simulink model "InnerOuter_Sim"  (Simulink 6.6)
settings: Solver=ode4  StartTime=0.0  StopTime=125  FixedStep=SampleT  RelTol=1e-3
InitFcn:
  | clc
  | innerOuterInit
undefined symbols (not defined in the file): A1, Apolar, apSampleTime, bankCommandLimit, baseHeight, baseTemp, CD0, chord, CL0, CLa, CLa_dot, Clb, ClDa, CLDe, CLDf, ClDr, clock, Clp, CLq, Clr, Cm0, Cma, CmDe, CmDf, Cmq, Cnb, CnDa, CnDr, Cnp, Cnr, compensatorOn, CYb, CYDr, da_failamp, da_failbias, da_failper, daL_fail, daLimit, daR_fail, deg, deLimit, derivativesConstant, dr_fail, dr_failamp, dr_failbias, dr_failper, drLimit, dtLimit, Earth, elarm, Euler_0, F, gaind, getWP, ISA_g, Ixx, Iyy, Izz, L1OF, L2_base ... (+28)
libraries: simulink x102, SLUGS_Library x23, aerolibconvert2 x15, dsPICdrivers x8, aerolibactuator x5, aerolibtransform2 x2, aerolibwind2 x2, dspmtrx3 x2, aerolibatmos2 x1, aerolibutil x1
(part 2 of 4)

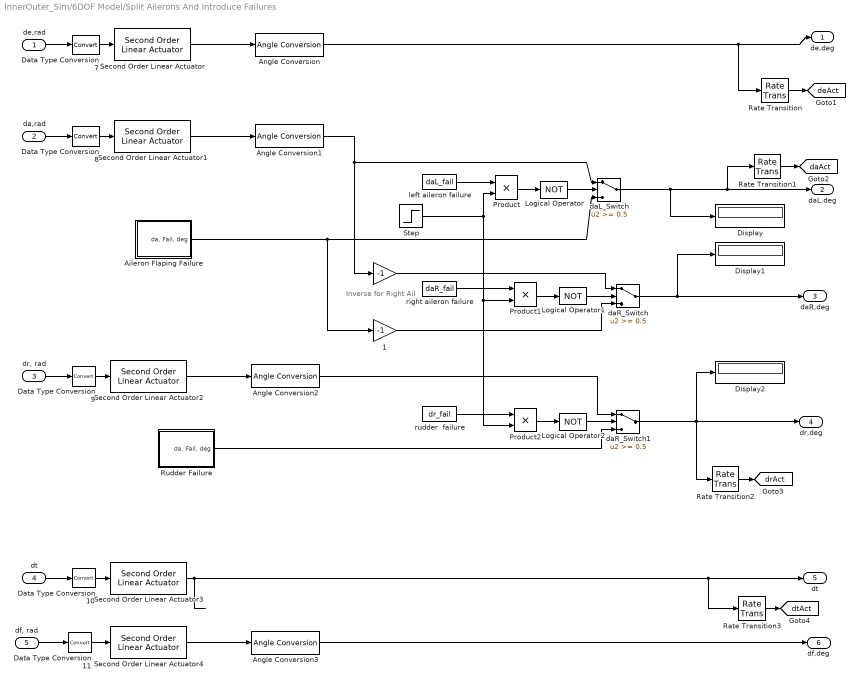
== system InnerOuter_Sim/6DOF Model/Split Ailerons And Introduce Failures ==
  note: Inverse
      | for Right
      | Ail
  de,rad : Inport
  da,rad : Inport  Port=2
  "dr, rad" : Inport  Port=3
  dt : Inport  Port=4
  "df, rad" : Inport  Port=5
  " " : Gain  Gain=-1  SaturateOnIntegerOverflow=on
  " 1" : Gain  Gain=-1  SaturateOnIntegerOverflow=on
  Aileron Flaping Failure : Subsystem
  Angle Conversion{,1..3} (4 alike) : aerolibconvert2/Angle Conversion  SystemSampleTime=-1  IU=rad  OU=deg
  Data Type Conversion{7..11} (5 alike) : DataTypeConversion  OutDataTypeMode=double
  Display : Display
  Display1 : Display
  Display2 : Display
  Logical Operator : Logic  Operator=NOT  AllPortsSameDT=off  OutDataTypeMode=Boolean
  Logical Operator1 : Logic  Operator=NOT  AllPortsSameDT=off  OutDataTypeMode=Boolean
  Logical Operator2 : Logic  Operator=NOT  AllPortsSameDT=off  OutDataTypeMode=Boolean
  Product : Product  RndMeth=Zero
  Product1 : Product  RndMeth=Zero
  Product2 : Product  RndMeth=Zero
  Rate Transition{,1..3} (4 alike) : RateTransition  OutPortSampleTime=apSampleTime
  Rudder Failure : Subsystem
  Second Order Linear Actuator{,1..3} (4 alike) : aerolibactuator/Second Order Linear Actuator  SystemSampleTime=-1  wn_fin=15  z_fin=0.8  fin_act_0=0
  Second Order Linear Actuator4 : aerolibactuator/Second Order Linear Actuator  SystemSampleTime=-1  wn_fin=150  z_fin=0.7  fin_act_0=0
  Step : Step  Time=tfailure
  daL_Switch : Switch  Threshold=0.5
  daR_Switch : Switch  Threshold=0.5
  daR_Switch1 : Switch  Threshold=0.5
  left aileron failure : Constant  Value=daL_fail
  right aileron failure : Constant  Value=daR_fail
  rudder  failure : Constant  Value=dr_fail
  de,deg : Outport
  daL,deg : Outport  Port=2
  daR,deg : Outport  Port=3
  dr,deg : Outport  Port=4
  "dt " : Outport  Port=5
  df,deg : Outport  Port=6
  tag scope: daAct=global, deAct=global, drAct=global, dtAct=global
  wires:
  de,rad/1 -> Data Type Conversion7/1
  da,rad/1 -> Data Type Conversion8/1
  "dr, rad"/1 -> Data Type Conversion9/1
  dt/1 -> Data Type Conversion10/1
  "df, rad"/1 -> Data Type Conversion11/1
  Second Order Linear Actuator/1 -> Angle Conversion/1
  Second Order Linear Actuator1/1 -> Angle Conversion1/1
  Second Order Linear Actuator2/1 -> Angle Conversion2/1
  Second Order Linear Actuator3/1 -> "dt "/1, Rate Transition3/1
  Second Order Linear Actuator4/1 -> Angle Conversion3/1
  Rate Transition1/1 -> [daAct]
  Rate Transition2/1 -> [drAct]
  Rate Transition3/1 -> [dtAct]
  Data Type Conversion7/1 -> Second Order Linear Actuator/1
  Data Type Conversion8/1 -> Second Order Linear Actuator1/1
  Data Type Conversion9/1 -> Second Order Linear Actuator2/1
  Data Type Conversion10/1 -> Second Order Linear Actuator3/1
  Data Type Conversion11/1 -> Second Order Linear Actuator4/1
  Angle Conversion/1 -> de,deg/1, Rate Transition/1
  Angle Conversion1/1 -> daL_Switch/1, " "/1
  Angle Conversion2/1 -> daR_Switch1/1
  Angle Conversion3/1 -> df,deg/1
  left aileron failure/1 -> Product/1
  Aileron Flaping Failure/1("da, Fail, deg") -> daL_Switch/3, " 1"/1
  Product/1 -> Logical Operator/1
  Logical Operator/1 -> daL_Switch/2
  Step/1 -> Product/2, Product1/2, Product2/2
  daL_Switch/1 -> Display/1, daL,deg/1, Rate Transition1/1
  right aileron failure/1 -> Product1/1
  Product1/1 -> Logical Operator1/1
  Logical Operator1/1 -> daR_Switch/2
  " "/1 -> daR_Switch/1
  " 1"/1 -> daR_Switch/3
  daR_Switch/1 -> daR,deg/1, Display1/1
  rudder  failure/1 -> Product2/1
  Product2/1 -> Logical Operator2/1
  Logical Operator2/1 -> daR_Switch1/2
  daR_Switch1/1 -> dr,deg/1, Display2/1, Rate Transition2/1
  Rate Transition/1 -> [deAct]
  Rudder Failure/1("da, Fail, deg") -> daR_Switch1/3

== system InnerOuter_Sim/6DOF Model/Subsystem ==
  Signal In : Inport  Orientation=down
  Noise On : Inport  Port=2
  Add : Sum  OutScaling=2^-10
  Random Number : RandomNumber  Variance=nv  Seed=ns  SampleTime=st
  Signal1 : InportShadow  Port=1  LatchByCopyingInsideSignal=off
  Switch : Switch  Threshold=0.3
  Signal Out : Outport
  wires:
  Random Number/1 -> Add/2
  Add/1 -> Switch/1
  Signal In/1 -> Add/1
  Noise On/1 -> Switch/2
  Switch/1 -> Signal Out/1
  Signal1/1 -> Switch/3

== system InnerOuter_Sim/6DOF Model/Subsystem1 ==
  Signal In : Inport  Orientation=down
  Noise On : Inport  Port=2
  Add : Sum  OutScaling=2^-10
  Random Number : RandomNumber  Variance=nv  Seed=ns  SampleTime=st
  Signal1 : InportShadow  Port=1  LatchByCopyingInsideSignal=off
  Switch : Switch  Threshold=0.3
  Signal Out : Outport
  wires:
  Signal1/1 -> Switch/3
  Switch/1 -> Signal Out/1
  Noise On/1 -> Switch/2
  Signal In/1 -> Add/1
  Add/1 -> Switch/1
  Random Number/1 -> Add/2

== system InnerOuter_Sim/6DOF Model/Subsystem2 ==
  Signal In : Inport  Orientation=down
  Noise On : Inport  Port=2
  Add : Sum  OutScaling=2^-10
  Random Number : RandomNumber  Variance=nv  Seed=ns  SampleTime=st
  Signal1 : InportShadow  Port=1  LatchByCopyingInsideSignal=off
  Switch : Switch  Threshold=0.3
  Signal Out : Outport
  wires:
  Random Number/1 -> Add/2
  Add/1 -> Switch/1
  Signal In/1 -> Add/1
  Noise On/1 -> Switch/2
  Switch/1 -> Signal Out/1
  Signal1/1 -> Switch/3

== system InnerOuter_Sim/6DOF Model/Subsystem3 ==
  Signal In : Inport  Orientation=down
  Noise On : Inport  Port=2
  Add : Sum  OutScaling=2^-10
  Random Number : RandomNumber  Variance=nv  Seed=ns  SampleTime=st
  Signal1 : InportShadow  Port=1  LatchByCopyingInsideSignal=off
  Switch : Switch  Threshold=0.3
  Signal Out : Outport
  wires:
  Signal1/1 -> Switch/3
  Switch/1 -> Signal Out/1
  Noise On/1 -> Switch/2
  Signal In/1 -> Add/1
  Add/1 -> Switch/1
  Random Number/1 -> Add/2

== system InnerOuter_Sim/6DOF Model/Subsystem4 ==
  Signal In : Inport  Orientation=down
  Noise On : Inport  Port=2
  Add : Sum  OutScaling=2^-10
  Random Number : RandomNumber  Variance=nv  Seed=ns  SampleTime=st
  Signal1 : InportShadow  Port=1  LatchByCopyingInsideSignal=off
  Switch : Switch  Threshold=0.3
  Signal Out : Outport
  wires:
  Signal1/1 -> Switch/3
  Switch/1 -> Signal Out/1
  Noise On/1 -> Switch/2
  Signal In/1 -> Add/1
  Add/1 -> Switch/1
  Random Number/1 -> Add/2

== system InnerOuter_Sim/6DOF Model/Subsystem5 ==
  Signal In : Inport  Orientation=down
  Noise On : Inport  Port=2
  Add : Sum  OutScaling=2^-10
  Random Number : RandomNumber  Variance=nv  Seed=ns  SampleTime=st
  Signal1 : InportShadow  Port=1  LatchByCopyingInsideSignal=off
  Switch : Switch  Threshold=0.3
  Signal Out : Outport
  wires:
  Random Number/1 -> Add/2
  Add/1 -> Switch/1
  Signal In/1 -> Add/1
  Noise On/1 -> Switch/2
  Switch/1 -> Signal Out/1
  Signal1/1 -> Switch/3

== system InnerOuter_Sim/6DOF Model/Subsystem6 ==
  Signal In : Inport  Orientation=down
  Noise On : Inport  Port=2
  Add : Sum  OutScaling=2^-10
  Random Number : RandomNumber  Variance=nv  Seed=ns  SampleTime=st
  Signal1 : InportShadow  Port=1  LatchByCopyingInsideSignal=off
  Switch : Switch  Threshold=0.3
  Signal Out : Outport
  wires:
  Signal1/1 -> Switch/3
  Switch/1 -> Signal Out/1
  Noise On/1 -> Switch/2
  Signal In/1 -> Add/1
  Add/1 -> Switch/1
  Random Number/1 -> Add/2

== system InnerOuter_Sim/BaroTest/Compute Barometric Height ==
  Base Height (m) : Inport
  Base Pressure (Pa) : Inport  Port=2
  Baro (Pa) : Inport  Port=3
  Constant2 : Constant  Value=baseTemp/(-LapseRate)  OutDataTypeMode=single
  Constant3 : Constant  Value=9.350253e-2  OutDataTypeMode=single
  Constant4 : Constant  Value=-1.888933e-1  OutDataTypeMode=single
  Constant5 : Constant  Value=2.180313e-5  OutDataTypeMode=single
  Divide : Product  Inputs=*/  OutDataTypeMode=single  OutScaling=2^-10
  Divide{1..4} (4 alike) : Product  OutDataTypeMode=single  OutScaling=2^-10
  Length Conversion : aerolibconvert2/Length Conversion  SystemSampleTime=-1  IU=ft  OU=m
  Sum1 : Sum  Inputs=|++  OutDataTypeMode=single
  Sum2 : Sum  Inputs=|+-  OutDataTypeMode=single
  Sum3 : Sum  Inputs=3  OutDataTypeMode=single
  "Altitude, m" : Outport
  wires:
  Length Conversion/1 -> Sum1/1
  Sum2/1 -> Divide/1
  Sum1/1 -> "Altitude, m"/1
  Divide3/1 -> Length Conversion/1
  Constant2/1 -> Divide3/2
  Sum3/1 -> Divide3/1
  Constant5/1 -> Sum3/3
  Divide2/1 -> Sum3/2
  Divide1/1 -> Sum3/1
  Constant4/1 -> Divide2/2
  Constant3/1 -> Divide1/2
  Divide4/1 -> Divide1/1  "x^2"
  Divide/1 -> Divide2/1, Divide4/1, Divide4/2  "x"
  Base Pressure (Pa)/1 -> Divide/2, Sum2/2
  Base Height (m)/1 -> Sum1/2
  Baro (Pa)/1 -> Sum2/1

== system InnerOuter_Sim/BaroTest/Initial Baro Bias ==
  Baro (Pa) : Inport
  Enable : EnablePort
  Data Type Conversion : DataTypeConversion  OutDataTypeMode=double
  Data Type Conversion1 : DataTypeConversion  OutDataTypeMode=single
  Low Pass8 : Subsystem  mask(DiscretizedZeroPole){Zeros=[], Poles=[-3], Gain=3, AbsTol=auto, SampleTime=.01, method=tustin, Wc=1}
      mask prompts: Zeros "Zeros (enter in s-main:)"; Poles "Poles (enter in s-domain:)"; Gain "Gain (enter in s-domain:)"; AbsTol "Absolute tolerance:"; SampleTime "Sample time:"; Wc "Critical Frequency (Hz):"
      mask help: Continuous mask uses c2d to transform parameters onto the Discrete Zero-Pole block inside.
      mask init:
      | st=SampleTime;
      | if length(st)>1
      |     st=SampleTime(1);
      | end
      | if(st>0)
      |     [zerosd,polesd,gaind] = sldiscutil('disczpk', {st,method,Wc,Zeros,Poles,Gain});
      | end	
      | s = get_param(gcb,'maskvalues');
      | zeross = s{1};
      | poless = s{2};
      | gainss = s{3};
      | %zerosc = eval(zeross);
      | %polesc = eval(poless);
      | %gainsc = eval(gainss);
      | sldiscutil('initzpkmask', st);
      | if(st==0)
      | set_param([gcb '/Zero Pole'], 'AbsoluteTolerance', AbsTol);
      | end
      mask StyleString: edit,edit,edit,edit,edit,popup(zoh|foh|tustin|prewarp|matched),edit
      mask CallbackString: |||||hidecrit|
      mask Display:
      | droots(zeross,poless,gainss)
      | text( 0.5, 1.0, method, 'verticalAlignment','top')
  Mux : Mux  Inputs=2
  Scope : Scope
      settings: SaveName=ScopeData8
  "[80k - 120k]" : Saturate  UpperLimit=120000  LowerLimit=80000
  Baro (Gnd) : Outport
  wires:
  Baro (Pa)/1 -> Data Type Conversion/1
  Low Pass8/1(Out1) -> Data Type Conversion1/1
  Data Type Conversion/1 -> Low Pass8/1(In1)
  Data Type Conversion1/1 -> Mux/2, "[80k - 120k]"/1
  Mux/1 -> Scope/1
  "[80k - 120k]"/1 -> Baro (Gnd)/1, Mux/1

== system InnerOuter_Sim/BaroTest/Zero Out Height ==
  Base Height : Inport
  Computed Height : Inport  Port=2
  Enable : EnablePort
  Integer Delay : simulink/Discrete/Integer Delay  vinit=0  samptime=.01  NumDelays=1
  Sum : Sum  Inputs=|+-  OutDataTypeMode=single
  Height Offset : Outport
  wires:
  Computed Height/1 -> Integer Delay/1
  Sum/1 -> Height Offset/1
  Integer Delay/1 -> Sum/2
  Base Height/1 -> Sum/1

== system InnerOuter_Sim/Compute psi_dot_m/Subsystem5 ==
  u : Inport
  C Function Call1 : dsPICdrivers/OTHERS/C Function Call  Tag=dsPIC_dsPIC_CFunctionCall  fctName='myCos'  INPUT_SIZE=1  INPUT1=real32  INPUT2=--  INPUT3=--  OUTPUT_SIZE=1  OUTPUT1=real32  SampleTime=-1  InputType=[ 7 ]  OutputType=[ 7 ]  FctDeclaration=extern real32_T myCos(real32_T u1);  FctCall=%y1 = myCos(%u1);  OrderingInOutPopup=None
  Environment Controller1 : simulink/Signal Routing/Environment Controller  SystemSampleTime=-1
  Trigonometric Function : Trigonometry  Operator=cos
  cos(u) : Outport
  wires:
  u/1 -> C Function Call1/1, Trigonometric Function/1
  Environment Controller1/1 -> cos(u)/1
  C Function Call1/1 -> Environment Controller1/2
  Trigonometric Function/1 -> Environment Controller1/1

== system InnerOuter_Sim/L1 Output Feedback Controller With  Projection Operator/Control  Law ==
  a : Inport
  u : Inport  Port=2
  Compute Coef : Subsystem
  Detect Change : Subsystem
  Divide : Product  OutScaling=2^-10  SampleTime=apSampleTime
  Divide1 : Product  OutScaling=2^-10  SampleTime=apSampleTime
  IC : InitialCondition
  Integer Delay : simulink/Discrete/Integer Delay  vinit=0.0  samptime=apSampleTime  NumDelays=1
  Integer Delay1 : simulink/Discrete/Integer Delay  Orientation=left  vinit=0.0  samptime=apSampleTime  NumDelays=1
  Subtract : Sum  OutScaling=2^-10  SampleTime=apSampleTime
  y : Outport
  wires:
  Integer Delay1/1 -> Divide1/2
  u/1 -> Integer Delay/1
  IC/1 -> Compute Coef/Enable
  Subtract/1 -> Integer Delay1/1, y/1
  Divide1/1 -> Subtract/2
  Divide/1 -> Subtract/1
  Integer Delay/1 -> Divide/2
  Detect Change/1(change?) -> IC/1
  Compute Coef/2(c) -> Divide1/1
  Compute Coef/1(b) -> Divide/1
  a/1 -> Detect Change/1(Data), Compute Coef/1(a)

== system InnerOuter_Sim/L1 Output Feedback Controller With  Projection Operator/Projection Operator ==
  Theta Max : Inport
  Eps 0 : Inport  Port=2
  Theta : Inport  Port=3
  y : Inport  Port=4
  Compare To Zero : simulink/Logic and Bit Operations/Compare To Zero  SystemSampleTime=-1  relop=>=  LogicOutDataTypeMode=boolean  ZeroCross=off
  Compare To Zero1 : simulink/Logic and Bit Operations/Compare To Zero  SystemSampleTime=-1  relop=>  LogicOutDataTypeMode=boolean  ZeroCross=off
  Data Type Conversion1 : DataTypeConversion  OutDataType=fixdt(1, 16)
  Divide2 : Product  OutDataTypeMode=single  OutScaling=2^-10
  Enabled Subsystem : Subsystem  TreatAsAtomicUnit=on
  Enabled Subsystem1 : Subsystem  TreatAsAtomicUnit=on
  Enabled Subsystem2 : Subsystem  TreatAsAtomicUnit=on
  F(theta) : Subsystem
  Logical Operator : Logic  Operator=NOT  AllPortsSameDT=off  OutDataTypeMode=Specify via dialog
  Logical Operator2 : Logic  Orientation=down  AllPortsSameDT=off  OutDataTypeMode=Specify via dialog
  Merge : Merge  InitialOutput=0
  Scope1 : Scope  NumInputPorts=4
      settings: YMin=-0.6~-0.5~-100~-10  YMax=0~5~10~10  SaveName=ScopeData4
  Scope2 : Scope  NumInputPorts=2
      settings: TimeRange=400  YMin=-0.06~-0.06  YMax=0.06~0.06  SaveName=ScopeData15
  "y " : InportShadow  Port=4  LatchByCopyingInsideSignal=off
  "y    " : InportShadow  Port=4  LatchByCopyingInsideSignal=off
  "Proj(the, y)" : Outport
  wires:
  Enabled Subsystem1/1(Out1) -> Merge/2
  "y    "/1 -> Enabled Subsystem1/1(y), Enabled Subsystem2/1(y), Scope1/2
  Logical Operator/1 -> Enabled Subsystem/Enable, Scope2/2
  Logical Operator2/1 -> Logical Operator/1, Enabled Subsystem1/Enable, Enabled Subsystem2/Enable, Scope2/1
  Compare To Zero1/1 -> Logical Operator2/1
  F(theta)/2(dif_f_theta) -> Divide2/1, Enabled Subsystem1/3(grad), Enabled Subsystem2/3(grad), Scope1/4
  Compare To Zero/1 -> Logical Operator2/2
  Enabled Subsystem/1(Out1) -> Data Type Conversion1/1
  "y "/1 -> Enabled Subsystem/1(In1)
  Merge/1 -> "Proj(the, y)"/1
  Divide2/1 -> Compare To Zero1/1
  y/1 -> Divide2/2
  F(theta)/1(f_theta) -> Compare To Zero/1, Enabled Subsystem1/2(f_the), Enabled Subsystem2/2(f_the), Scope1/3
  Theta/1 -> F(theta)/3(Theta)
  Eps 0/1 -> F(theta)/2(Eps 0)
  Theta Max/1 -> F(theta)/1(Theta Max)
  Data Type Conversion1/1 -> Merge/1
  Enabled Subsystem2/1(Out1) -> Scope1/1

== system InnerOuter_Sim/L1 Output Feedback Controller With  Projection Operator/State Predictor ==
  a : Inport
  u : Inport  Port=2
  Compute Coef : Subsystem
  Detect Change : Subsystem
  Divide : Product  OutScaling=2^-10  SampleTime=apSampleTime
  Divide1 : Product  OutScaling=2^-10  SampleTime=apSampleTime
  IC : InitialCondition
  Integer Delay : simulink/Discrete/Integer Delay  vinit=0.0  samptime=apSampleTime  NumDelays=1
  Integer Delay1 : simulink/Discrete/Integer Delay  Orientation=left  vinit=0.0  samptime=apSampleTime  NumDelays=1
  Subtract : Sum  OutScaling=2^-10  SampleTime=apSampleTime
  y : Outport
  wires:
  a/1 -> Compute Coef/1(a), Detect Change/1(Data)
  Compute Coef/1(b) -> Divide/1
  Compute Coef/2(c) -> Divide1/1
  Detect Change/1(change?) -> IC/1
  Integer Delay/1 -> Divide/2
  Divide/1 -> Subtract/1
  Divide1/1 -> Subtract/2
  Subtract/1 -> y/1, Integer Delay1/1
  IC/1 -> Compute Coef/Enable
  u/1 -> Integer Delay/1
  Integer Delay1/1 -> Divide1/2

== system InnerOuter_Sim/L1 Output Feedback Controller With  Projection Operator/Trapezoidal Integrator ==
  x : Inport
  Reset : Inport  Port=2
  Constant : Constant  Value=1/3  OutDataTypeMode=single
  Constant1 : Constant  Value=4/3  OutDataTypeMode=single
  Constant2 : Constant  Value=T/2  OutDataTypeMode=single
  Constant3 : Constant  Value=1/3  OutDataTypeMode=single
  Constant5 : Constant  Orientation=left  Value=0  OutDataTypeMode=single
  Integer Delay : simulink/Discrete/Integer Delay  vinit=0.0  samptime=T  NumDelays=1
  Integer Delay1 : simulink/Discrete/Integer Delay  vinit=0.0  samptime=T  NumDelays=2
  Integer Delay2 : simulink/Discrete/Integer Delay  Orientation=left  vinit=0.0  samptime=T  NumDelays=1
  Product{,1..3} (4 alike) : Product  OutDataTypeMode=single  RndMeth=Zero
  Protect NaNs : Subsystem
  Protect NaNs1 : Subsystem
  Subtract : Sum  Inputs=3  OutDataTypeMode=single  OutScaling=2^-10
  Subtract1 : Sum  Inputs=2  OutDataTypeMode=single  OutScaling=2^-10
  Switch1 : Switch  Criteria=u2 > Threshold  Threshold=0.3  SampleTime=.01
  "[min max]" : Saturate  UpperLimit=upperLimit  LowerLimit=lowerLimit  SampleTime=T
  Int(x) : Outport
  wires:
  Protect NaNs1/1(Out1) -> Integer Delay2/1, Int(x)/1
  Protect NaNs/1(Out1) -> Integer Delay1/1, Integer Delay/1, Product/1
  Subtract1/1 -> "[min max]"/1
  Product3/1 -> Subtract1/2
  "[min max]"/1 -> Switch1/3
  Switch1/1 -> Protect NaNs1/1(In1)
  Reset/1 -> Switch1/2
  Constant5/1 -> Switch1/1
  Integer Delay2/1 -> Subtract1/1
  Subtract/1 -> Product3/2
  Constant2/1 -> Product3/1
  Product2/1 -> Subtract/3
  Product1/1 -> Subtract/2
  Product/1 -> Subtract/1
  x/1 -> Protect NaNs/1(In1)
  Constant3/1 -> Product2/2
  Integer Delay1/1 -> Product2/1
  Integer Delay/1 -> Product1/1
  Constant1/1 -> Product1/2
  Constant/1 -> Product/2

== system InnerOuter_Sim/Lateral Channel/0.5 sec  tau ==
  In1 : Inport
  Constant : Constant  Value=T
  Constant1 : Constant  Value=f
  Embedded MATLAB Function : Stateflow chart
  Out1 : Outport
  wires:
  In1/1 -> Embedded MATLAB Function/1(u)
  Embedded MATLAB Function/1(y) -> Out1/1
  Constant1/1 -> Embedded MATLAB Function/3(f)
  Constant/1 -> Embedded MATLAB Function/2(T)

== system InnerOuter_Sim/Lateral Channel/Bank to Psi Dot ==
  phi_c : Inport
  U_m : Inport  Port=2
  Constant1 : Constant  Value=9.80665  OutDataTypeMode=single
  Divide : Product  Inputs=/*  OutDataTypeMode=single  OutScaling=2^-10  SampleTime=apSampleTime
  Divide1 : Product  OutDataTypeMode=single  OutScaling=2^-10  SampleTime=apSampleTime
  Subsystem8 : SLUGS_Library/Subsystem8  SystemSampleTime=-1
  negprotect : Stateflow chart
  psi_dot_c : Outport
  wires:
  negprotect/1(zpVal) -> Divide/1
  Divide/1 -> Divide1/2
  phi_c/1 -> Subsystem8/1
  Subsystem8/1 -> Divide1/1
  Divide1/1 -> psi_dot_c/1
  Constant1/1 -> Divide/2
  U_m/1 -> negprotect/1(val)

== system InnerOuter_Sim/Lateral Channel/Sideslip Compensation ==
  phi_m : Inport
  r_m : Inport  Port=2
  U_m : Inport  Port=3
  Enable : EnablePort  StatesWhenEnabling=reset
  Bank to Psi Dot : Subsystem  AncestorBlock=SLUGS_Library/Navigation/Bank to Psi Dot
  Constant : Constant  Value=0.3  OutDataTypeMode=single
  Low Pass : Subsystem
      mask Display:
      | droots([],'-a','a')
      | port_label('input',1,'a')
      | port_label('input',2,'u')
      | port_label('output',1,'y')
  Subtract : Sum  Inputs=+-  OutScaling=2^-10
  psi_dot to Bank : Subsystem  AncestorBlock=SLUGS_Library/Navigation/psi_dot to Bank
  bankComp : Outport  OutputWhenDisabled=reset  InitialOutput=0
  wires:
  phi_m/1 -> Bank to Psi Dot/1(phi_c)
  r_m/1 -> Subtract/2
  U_m/1 -> Bank to Psi Dot/2(U_m), psi_dot to Bank/2(U_m)
  Bank to Psi Dot/1(psi_dot_c) -> Subtract/1  "coord turn"
  Subtract/1 -> psi_dot to Bank/1(psi_dot_c)  "turn rate error"
  psi_dot to Bank/1(phi_c) -> Low Pass/2(u)  "phi error"
  Low Pass/1(y) -> bankComp/1
  Constant/1 -> Low Pass/1(a)

== system InnerOuter_Sim/Lateral Channel/psi_dot to Bank ==
  psi_dot_c : Inport
  U_m : Inport  Port=2
  Constant1 : Constant  Value=9.80665  OutDataTypeMode=single
  Divide : Product  Inputs=**/  OutScaling=2^-10  SampleTime=apSampleTime
  Subsystem2 : SLUGS_Library/Subsystem2  SystemSampleTime=-1
  phi_c : Outport
  wires:
  Divide/1 -> Subsystem2/1
  Subsystem2/1 -> phi_c/1
  Constant1/1 -> Divide/3
  U_m/1 -> Divide/2
  psi_dot_c/1 -> Divide/1

== system InnerOuter_Sim/Longitudinal Channel/0.3 sec  tau for low speeds ==
  In1 : Inport
  Constant : Constant  Value=T
  Constant1 : Constant  Value=f
  Embedded MATLAB Function : Stateflow chart
  Out1 : Outport
  wires:
  In1/1 -> Embedded MATLAB Function/1(u)
  Embedded MATLAB Function/1(y) -> Out1/1
  Constant1/1 -> Embedded MATLAB Function/3(f)
  Constant/1 -> Embedded MATLAB Function/2(T)

== system InnerOuter_Sim/Longitudinal Channel/0.5 sec  tau for Turns ==
  In1 : Inport
  Constant : Constant  Value=T
  Constant1 : Constant  Value=f
  Embedded MATLAB Function : Stateflow chart
  Out1 : Outport
  wires:
  In1/1 -> Embedded MATLAB Function/1(u)
  Embedded MATLAB Function/1(y) -> Out1/1
  Constant1/1 -> Embedded MATLAB Function/3(f)
  Constant/1 -> Embedded MATLAB Function/2(T)

== system InnerOuter_Sim/Longitudinal Channel/5 sec tau for high speeds ==
  In1 : Inport
  Constant : Constant  Value=T
  Constant1 : Constant  Value=f
  Embedded MATLAB Function : Stateflow chart
  Out1 : Outport
  wires:
  In1/1 -> Embedded MATLAB Function/1(u)
  Embedded MATLAB Function/1(y) -> Out1/1
  Constant1/1 -> Embedded MATLAB Function/3(f)
  Constant/1 -> Embedded MATLAB Function/2(T)

== system InnerOuter_Sim/Longitudinal Channel/Air Density from Height ==
  h(m) : Inport
  Add : Sum  Inputs=+-  OutScaling=2^-10
  Constant : Constant  OutDataTypeMode=single
  Constant 2 from Model : Constant  Value=4.255876  OutDataTypeMode=single
  Constant from Model : Constant  Value=145442  OutDataTypeMode=single
  Divide : Product  Inputs=*/  OutScaling=2^-10  SampleTime=.01
  Divide1 : Product  OutScaling=2^-10
  Length Conversion : aerolibconvert2/Length Conversion  SystemSampleTime=-1  IU=m  OU=ft
  Rho_0 (Kg/m^3) : Constant  Value=1.225  OutDataTypeMode=single
  Subsystem : SLUGS_Library/Subsystem  SystemSampleTime=-1
  rho (Kg/m^3) : Outport
  wires:
  Constant/1 -> Add/1
  Divide/1 -> Add/2
  h(m)/1 -> Length Conversion/1
  Constant from Model/1 -> Divide/2
  Rho_0 (Kg/m^3)/1 -> Divide1/2
  Divide1/1 -> rho (Kg/m^3)/1
  Length Conversion/1 -> Divide/1
  Add/1 -> Subsystem/1
  Constant 2 from Model/1 -> Subsystem/2
  Subsystem/1 -> Divide1/1

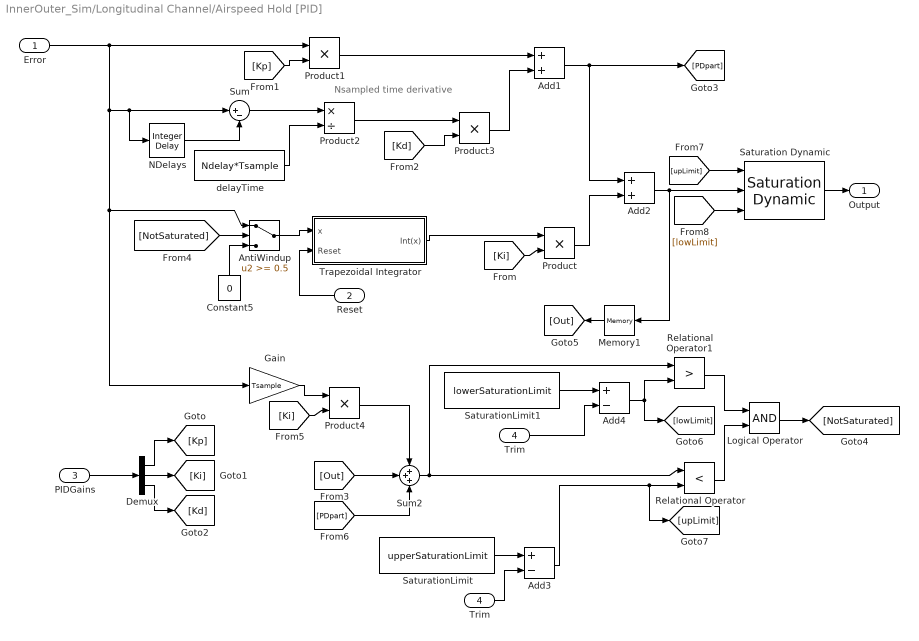
== system InnerOuter_Sim/Longitudinal Channel/Airspeed Hold [PID] ==
  note: Nsampled time derivative
  Error : Inport
  Reset : Inport  Orientation=left  Port=2
  PIDGains : Inport  Port=3
  Trim : Inport  Port=4
  Add1 : Sum  OutScaling=2^-10
  Add2 : Sum  OutDataTypeMode=single  OutScaling=2^-10
  Add3 : Sum  Inputs=+-  OutDataTypeMode=single  OutScaling=2^-10
  Add4 : Sum  Inputs=+-  OutDataTypeMode=single  OutScaling=2^-10
  AntiWindup : Switch  Threshold=0.5
  Constant5 : Constant  Orientation=up  Value=0  OutDataTypeMode=double
  Demux : Demux  Outputs=3
  Gain : Gain  Gain=Tsample
  Logical Operator : Logic  AllPortsSameDT=off  OutDataTypeMode=Boolean
  Memory1 : Memory  Orientation=left  InheritSampleTime=on
  NDelays : simulink/Discrete/Integer Delay  vinit=0.0  samptime=Tsample  NumDelays=Ndelay
  Product{,1,3..4} (4 alike) : Product  RndMeth=Zero
  Product2 : Product  Inputs=*/  RndMeth=Zero
  Relational Operator : RelationalOperator  Operator=<  LogicOutDataTypeMode=Boolean
  Relational Operator1 : RelationalOperator  Operator=>  LogicOutDataTypeMode=Boolean
  Saturation Dynamic : simulink/Discontinuities/Saturation Dynamic  SystemSampleTime=-1
  SaturationLimit : Constant  Value=upperSaturationLimit  OutDataTypeMode=single
  SaturationLimit1 : Constant  Value=lowerSaturationLimit  OutDataTypeMode=single
  Sum : Sum  Inputs=|+-
  Sum2 : Sum  Inputs=+++
  Trapezoidal Integrator : Subsystem  mask{T=Tsample}
      mask prompts: T "Sample Time"
  "Trim " : InportShadow  Port=4  LatchByCopyingInsideSignal=off
  delayTime : Constant  Value=Ndelay*Tsample  OutDataTypeMode=single
  Output : Outport
  wires:
  [NotSaturated] -> AntiWindup/2
  Saturation Dynamic/1 -> Output/1
  Product2/1 -> Product3/1
  [Kd] -> Product3/2
  delayTime/1 -> Product2/2
  Sum/1 -> Product2/1
  NDelays/1 -> Sum/2
  Add2/1 -> Memory1/1, Saturation Dynamic/2
  [Kp] -> Product1/2
  Trapezoidal Integrator/1(Int(x)) -> Product/1
  [Ki] -> Product/2
  Error/1 -> Product1/1, Sum/1, NDelays/1, AntiWindup/1, Gain/1
  AntiWindup/1 -> Trapezoidal Integrator/1(x)
  Constant5/1 -> AntiWindup/3
  Demux/3 -> [Kd]
  Demux/2 -> [Ki]
  Demux/1 -> [Kp]
  PIDGains/1 -> Demux/1
  Memory1/1 -> [Out]
  Reset/1 -> Trapezoidal Integrator/2(Reset)
  Product1/1 -> Add1/1
  Product3/1 -> Add1/2
  Add1/1 -> [PDpart], Add2/1
  Product/1 -> Add2/2
  [PDpart] -> Sum2/3
  Product4/1 -> Sum2/1
  Gain/1 -> Product4/1
  [Ki] -> Product4/2
  Sum2/1 -> Relational Operator/1, Relational Operator1/1
  [Out] -> Sum2/2
  Add3/1 -> Relational Operator/2, [upLimit]
  Relational Operator/1 -> Logical Operator/2
  Relational Operator1/1 -> Logical Operator/1
  Logical Operator/1 -> [NotSaturated]
  Trim/1 -> Add3/2
  SaturationLimit/1 -> Add3/1
  Add4/1 -> Relational Operator1/2, [lowLimit]
  SaturationLimit1/1 -> Add4/1
  "Trim "/1 -> Add4/2
  [upLimit] -> Saturation Dynamic/1
  [lowLimit] -> Saturation Dynamic/3

== system InnerOuter_Sim/Longitudinal Channel/Compute Airspeed ==
  Dyn P : Inport
  rho : Inport  Port=2
  Divide2 : Product  Inputs=**/  OutScaling=2^-10  SampleTime=.01
  Subsystem1 : SLUGS_Library/Subsystem1  SystemSampleTime=-1
  "[ 0.01 50000]" : Saturate  UpperLimit=50000  LowerLimit=0.01
  a : Constant  Value=2  OutDataTypeMode=single
  Airspeed m(s) : Outport
  wires:
  "[ 0.01 50000]"/1 -> Divide2/3
  rho/1 -> "[ 0.01 50000]"/1
  Dyn P/1 -> Divide2/2
  a/1 -> Divide2/1
  Subsystem1/1 -> Airspeed m(s)/1
  Divide2/1 -> Subsystem1/1

== system InnerOuter_Sim/Longitudinal Channel/Subsystem5 ==
  u : Inport
  Trigonometric Function : Trigonometry  Operator=cos
  cos(u) : Outport
  wires:
  u/1 -> Trigonometric Function/1
  Trigonometric Function/1 -> cos(u)/1

== system InnerOuter_Sim/Navigation/Compute WP Switching Trigger ==
  Total Run : Inport
  T1 : Inport  Port=2
  WP0 : Inport  Port=3
  Puav : Inport  Port=4
  Compute  Projection : Subsystem
  Switch Distance Less than? : RelationalOperator  LogicOutDataTypeMode=Specify via dialog  SampleTime=apSampleTime
  Switch : Outport
  Tot Run : Outport  Port=2
  Dg : Outport  Port=3
  wires:
  Switch Distance Less than?/1 -> Switch/1
  T1/1 -> Compute  Projection/3(T)
  WP0/1 -> Compute  Projection/2(WP0)
  Puav/1 -> Compute  Projection/1(Puav)
  Total Run/1 -> Tot Run/1, Switch Distance Less than?/2
  Compute  Projection/1(Dg) -> Dg/1, Switch Distance Less than?/1

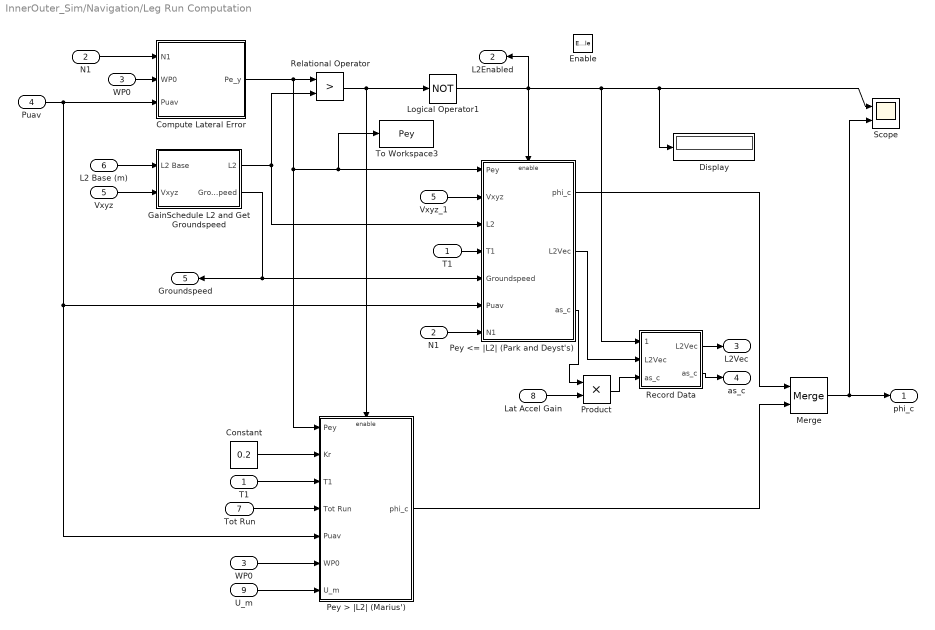
== system InnerOuter_Sim/Navigation/Leg Run Computation ==
  T1 : Inport
  N1 : Inport  Port=2
  WP0 : Inport  Port=3
  Puav : Inport  Port=4
  Vxyz : Inport  Port=5
  L2 Base (m) : Inport  Port=6
  Tot Run : Inport  Port=7
  Lat Accel Gain : Inport  Port=8
  U_m : Inport  Port=9
  Enable : EnablePort
  Compute Lateral Error : Subsystem  AncestorBlock=SLUGS_Library/Navigation/Compute Lateral Error
  Constant : Constant  Value=0.2  OutDataTypeMode=single
  Display : Display
  GainSchedule L2 and Get Groundspeed : Subsystem
  Logical Operator1 : Logic  Operator=NOT  AllPortsSameDT=off  OutDataTypeMode=Boolean
  Merge : Merge
  "N1 " : InportShadow  Port=2  LatchByCopyingInsideSignal=off
  Pey <= |L2| (Park and Deyst's) : Subsystem
  Pey > |L2| (Marius') : Subsystem
  Product : Product  RndMeth=Zero
  Record Data : Subsystem
  Relational Operator : RelationalOperator  Operator=>  LogicOutDataTypeMode=Boolean  ZeroCross=off
  Scope : Scope  NumInputPorts=2
      settings: YMin=0.95~-0.1  YMax=1.05~0.4  SaveName=ScopeData2
  "T1 " : InportShadow  Port=1  LatchByCopyingInsideSignal=off
  To Workspace3 : ToWorkspace  VariableName=Pey  SampleTime=-1  SaveFormat=Array
  Vxyz_1 : InportShadow  Port=5  LatchByCopyingInsideSignal=off
  "WP0 " : InportShadow  Port=3  LatchByCopyingInsideSignal=off
  phi_c : Outport
  L2Enabled : Outport  Orientation=left  Port=2
  L2Vec : Outport  Port=3
  as_c : Outport  Port=4
  Groundspeed : Outport  Orientation=left  Port=5
  wires:
  Compute Lateral Error/1(Pe_y) -> Relational Operator/1, Pey <= |L2| (Park and Deyst's)/1(Pey), To Workspace3/1, Pey > |L2| (Marius')/1(Pey)
  GainSchedule L2 and Get Groundspeed/1(L2) -> Relational Operator/2, Pey <= |L2| (Park and Deyst's)/3(L2)
  Vxyz/1 -> GainSchedule L2 and Get Groundspeed/2(Vxyz)
  L2 Base (m)/1 -> GainSchedule L2 and Get Groundspeed/1(L2 Base)
  Relational Operator/1 -> Logical Operator1/1, Pey > |L2| (Marius')/Enable
  Puav/1 -> Compute Lateral Error/3(Puav), Pey <= |L2| (Park and Deyst's)/6(Puav), Pey > |L2| (Marius')/5(Puav)
  GainSchedule L2 and Get Groundspeed/2(Groundspeed) -> Pey <= |L2| (Park and Deyst's)/5(Groundspeed), Groundspeed/1
  Vxyz_1/1 -> Pey <= |L2| (Park and Deyst's)/2(Vxyz)
  Logical Operator1/1 -> Pey <= |L2| (Park and Deyst's)/Enable, L2Enabled/1, Scope/1, Display/1, Record Data/1(ApMode)
  N1/1 -> Compute Lateral Error/1(N1)
  WP0/1 -> Compute Lateral Error/2(WP0)
  T1/1 -> Pey <= |L2| (Park and Deyst's)/4(T1)
  "N1 "/1 -> Pey <= |L2| (Park and Deyst's)/7(N1)
  Pey > |L2| (Marius')/1(phi_c) -> Merge/2
  "T1 "/1 -> Pey > |L2| (Marius')/3(T1)
  "WP0 "/1 -> Pey > |L2| (Marius')/6(WP0)
  Merge/1 -> phi_c/1, Scope/2
  Pey <= |L2| (Park and Deyst's)/1(phi_c) -> Merge/1
  Constant/1 -> Pey > |L2| (Marius')/2(Kr)
  Pey <= |L2| (Park and Deyst's)/2(L2Vec) -> Record Data/2("L2Vec ")
  Tot Run/1 -> Pey > |L2| (Marius')/4(Tot Run)
  Record Data/1(L2Vec) -> L2Vec/1
  Record Data/2("as_c ") -> as_c/1
  Product/1 -> Record Data/3(as_c)
  Pey <= |L2| (Park and Deyst's)/3(as_c) -> Product/1
  Lat Accel Gain/1 -> Product/2
  U_m/1 -> Pey > |L2| (Marius')/7(U_m)

== system InnerOuter_Sim/Navigation/Mode Determination ==
  Puav : Inport  SampleTime=apSampleTime
  WP Fly : Inport  Port=2
  Switch : Inport  Port=3
  Embedded MATLAB Function1 : Stateflow chart
  IC1 : InitialCondition
  Integer Delay6 : simulink/Discrete/Integer Delay  vinit=0  samptime=apSampleTime  NumDelays=1
  Logical Operator : Logic  Operator=OR  AllPortsSameDT=off  OutDataTypeMode=Boolean
  Recent Enable : Subsystem
  Switch Time Limit (in Samples) : Constant  Value=200  OutDataTypeMode=single
  Switch Mode : Outport
  WP Enabl : Outport  Port=2
  sw Increment : Outport  Port=3
  UAV IC : Outport  Port=4
  wires:
  Puav/1 -> Recent Enable/2(Puav)
  WP Fly/1 -> Recent Enable/1(WP Fly)
  Switch Time Limit (in Samples)/1 -> Embedded MATLAB Function1/2(timeLimit)
  Integer Delay6/1 -> Embedded MATLAB Function1/1(swDistanceRdy)
  Recent Enable/1(UAV IC) -> UAV IC/1
  Recent Enable/2(WPEnable) -> WP Enabl/1, Logical Operator/1
  Switch/1 -> Integer Delay6/1
  Embedded MATLAB Function1/1(swIncrement) -> Logical Operator/2, sw Increment/1
  Logical Operator/1 -> IC1/1
  IC1/1 -> Switch Mode/1

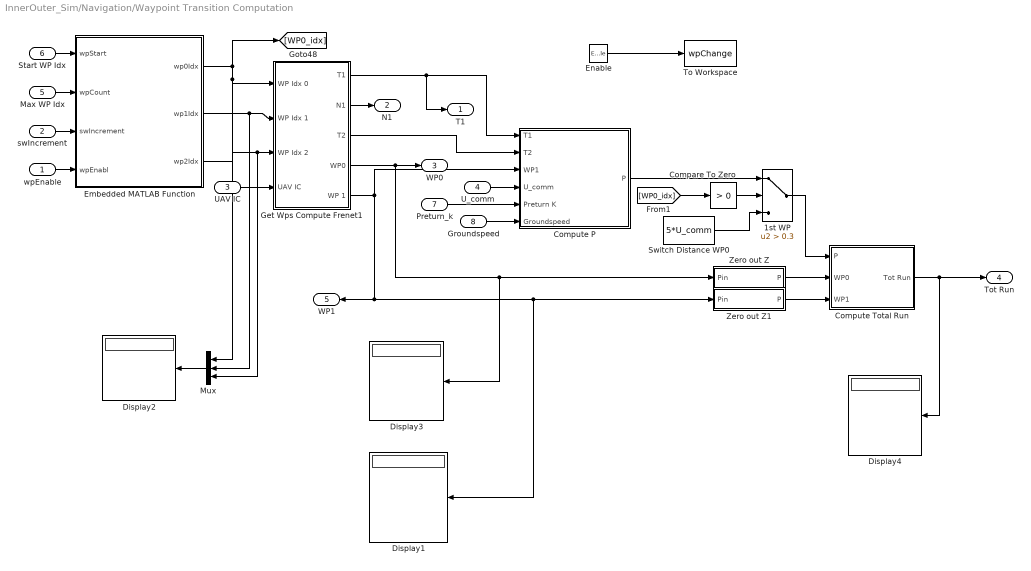
== system InnerOuter_Sim/Navigation/Waypoint Transition Computation ==
  wpEnable : Inport
  swIncrement : Inport  Port=2
  UAV IC : Inport  Port=3
  U_comm : Inport  Port=4
  Max WP Idx : Inport  Port=5
  Start WP Idx : Inport  Port=6
  Preturn_k : Inport  Port=7
  Groundspeed : Inport  Port=8
  Enable : EnablePort  ShowOutputPort=on
  1st WP : Switch  Criteria=u2 > Threshold  Threshold=0.3
  Compare To Zero : simulink/Logic and Bit Operations/Compare To Zero  SystemSampleTime=-1  relop=>  LogicOutDataTypeMode=uint8  ZeroCross=off
  Compute P : Subsystem
  Compute Total Run : Subsystem
  Display{1..4} (4 alike) : Display
  Embedded MATLAB Function : Stateflow chart
  Get Wps Compute Frenet1 : Subsystem
  Mux : Mux  Orientation=left  Inputs=3
  Switch Distance WP0 : Constant  Value=5*U_comm  OutDataTypeMode=single
  To Workspace : ToWorkspace  VariableName=wpChange  SampleTime=-1  SaveFormat=Structure
  Zero out Z : Stateflow chart
  Zero out Z1 : Stateflow chart
  T1 : Outport
  N1 : Outport  Port=2
  WP0 : Outport  Port=3
  Tot Run : Outport  Port=4
  WP1 : Outport  Orientation=left  Port=5
  wires:
  Start WP Idx/1 -> Embedded MATLAB Function/1(wpStart)
  Max WP Idx/1 -> Embedded MATLAB Function/2(wpCount)
  Embedded MATLAB Function/1(wp0Idx) -> [WP0_idx], Get Wps Compute Frenet1/1(WP Idx 0), Mux/1
  Embedded MATLAB Function/2(wp1Idx) -> Get Wps Compute Frenet1/2(WP Idx 1), Mux/2
  Embedded MATLAB Function/3(wp2Idx) -> Get Wps Compute Frenet1/3(WP Idx 2), Mux/3
  Get Wps Compute Frenet1/1(T1) -> Compute P/1(T1), T1/1
  Get Wps Compute Frenet1/3(T2) -> Compute P/2(T2)
  Get Wps Compute Frenet1/5(WP 1) -> WP1/1, Display1/1, Zero out Z1/1(Pin), Compute P/3(WP1)
  U_comm/1 -> Compute P/4(U_comm)
  Compute P/1(P) -> 1st WP/1
  Get Wps Compute Frenet1/2(N1) -> N1/1
  swIncrement/1 -> Embedded MATLAB Function/3(swIncrement)
  Get Wps Compute Frenet1/4(WP0) -> WP0/1, Display3/1, Zero out Z/1(Pin)
  wpEnable/1 -> Embedded MATLAB Function/4(wpEnabl)
  UAV IC/1 -> Get Wps Compute Frenet1/4(UAV IC)
  Enable/1 -> To Workspace/1
  Compute Total Run/1(Tot Run) -> Tot Run/1, Display4/1
  Compare To Zero/1 -> 1st WP/2
  Switch Distance WP0/1 -> 1st WP/3
  [WP0_idx] -> Compare To Zero/1
  1st WP/1 -> Compute Total Run/1(P)
  Mux/1 -> Display2/1
  Zero out Z/1(P) -> Compute Total Run/2("WP0  ")
  Zero out Z1/1(P) -> Compute Total Run/3(WP1)
  Preturn_k/1 -> Compute P/5(Preturn K)
  Groundspeed/1 -> Compute P/6(Groundspeed)

== system InnerOuter_Sim/6DOF Model/Plant/6-DOF EOM ==
  "[F,M]" : Inport
  Vb Corr : Inport  Orientation=left  Port=2
  Angular Rates : Integrator  InitialCondition=PQR_0'
  Demux1 : Demux  Outputs=2
  Euler Angles : Integrator  InitialCondition=Euler_0
  Get Euler Dot : Subsystem
      mask Display:
      | port_label('input', 1, 'p, q, r')
      | port_label('input', 2, 'Euler')
      | port_label('output', 1, 'Euler_dot')
  Mux : Mux  Orientation=left  Inputs=[3;3]
  NED2NEU : Gain  Gain=[1 0 0;0 1 0;0 0 -1]  Multiplication=Matrix(K*u)  SaturateOnIntegerOverflow=on
  Position : Integrator  InitialCondition=Pos_0'
  RB2L * Vb : Product  Multiplication=Matrix(*)  SaturateOnIntegerOverflow=on  InputSameDT=on
  RB2LTP : Subsystem
  Velocities Body : Integrator  InitialCondition=Vb_0'
  "[V1,2,3,W1,2,3]" : Subsystem
  X,Y,Z (LTP) : Outport
  "Vx, Vy, Vz" : Outport  Port=2
  Euler : Outport  Port=3
  "p, q, r" : Outport  Orientation=left  Port=4
  Vb : Outport  Port=5
  Ab meas : Outport  Port=6
  Euler_dot : Outport  Port=7
  wires:
  "[V1,2,3,W1,2,3]"/1("Acc_meas ") -> Ab meas/1
  Euler Angles/1 -> "[V1,2,3,W1,2,3]"/2(Euler), Get Euler Dot/2(Euler), Euler/1, RB2LTP/1(Euler)
  Demux1/1 -> Velocities Body/1
  "[V1,2,3,W1,2,3]"/2(V*dot) -> Demux1/1
  Demux1/2 -> Angular Rates/1
  "[F,M]"/1 -> "[V1,2,3,W1,2,3]"/1("[F ; M]")
  RB2LTP/1(Rot) -> RB2L * Vb/1
  Velocities Body/1 -> Vb/1, RB2L * Vb/2
  Mux/1 -> "[V1,2,3,W1,2,3]"/3(V*)
  Position/1 -> X,Y,Z (LTP)/1
  Angular Rates/1 -> Get Euler Dot/1(p,q,r), Mux/2, "p, q, r"/1
  RB2L * Vb/1 -> NED2NEU/1, "Vx, Vy, Vz"/1  "NED"
  NED2NEU/1 -> Position/1
  Get Euler Dot/1(Euler_dot) -> Euler Angles/1, Euler_dot/1
  Vb Corr/1 -> Mux/1

== system InnerOuter_Sim/6DOF Model/Plant/Engine Model ==
  dt : Inport
  Vmag : Inport  Port=2
  Constant4 : Constant  Value=0
  Get To1 : Subsystem
  Mux : Mux  Inputs=2
  Mux1 : Mux  Inputs=3
  Thrust Available (lbs) : Fcn  Expr=u(1) - 0.047*sqrt(u(1))*u(2)
  kg2N : Gain  Gain=ISA_g  SaturateOnIntegerOverflow=on
  lbs2kg : Gain  Gain=0.45359237  SaturateOnIntegerOverflow=on
  Thrust : Outport
  wires:
  dt/1 -> Get To1/1(dt)
  Get To1/1(To) -> Mux/1
  Mux/1 -> Thrust Available (lbs)/1
  Thrust Available (lbs)/1 -> lbs2kg/1
  Vmag/1 -> Mux/2
  Mux1/1 -> Thrust/1
  lbs2kg/1 -> kg2N/1
  Constant4/1 -> Mux1/2, Mux1/3
  kg2N/1 -> Mux1/1

== system InnerOuter_Sim/6DOF Model/Plant/Forces and Moments ==
  "Wind {E}" : Inport
  Rho : Inport  Port=2
  "de, deg" : Inport  Port=3
  daL,deg : Inport  Port=4
  daR,deg : Inport  Port=5
  "dr, deg" : Inport  Port=6
  "df, deg" : Inport  Port=7
  "Vx, Vy, Vz " : Inport  Port=8
  Euler : Inport  Port=9  PortDimensions=3
  p,q,r : Inport  Port=10
  Alpha/Beta : Subsystem
  Body Frame F & M : Subsystem
  Get Grav Force in Body : Subsystem
  Gravitational Force : Constant  Value=[0 0 mass*ISA_g]  VectorParams1D=off
  NED(u)2b : Subsystem
  Sum : Sum  Inputs=|++  SaturateOnIntegerOverflow=on
  Vair : Sum  Inputs=+-  SaturateOnIntegerOverflow=on  InputSameDT=on
  Airspeed : Outport
  Forces : Outport  Port=2
  Moments : Outport  Port=3
  Vb Corr : Outport  Port=4
  q : Outport  Port=5
  wires:
  Get Grav Force in Body/1(Grav Force (Body)) -> Sum/2
  Alpha/Beta/5(q) -> q/1
  "Vx, Vy, Vz "/1 -> Vair/1
  Vair/1 -> NED(u)2b/1(V w)
  Euler/1 -> NED(u)2b/2(Euler), Get Grav Force in Body/1(Euler)
  Rho/1 -> Alpha/Beta/2(Rho)
  NED(u)2b/1(Vb Corr) -> Alpha/Beta/1("Vx, Vy, Vz (Body)"), Vb Corr/1
  Body Frame F & M/2(M_b) -> Moments/1
  Gravitational Force/1 -> Get Grav Force in Body/2(Grav Force)
  Body Frame F & M/1(F_b) -> Sum/1
  Sum/1 -> Forces/1
  Alpha/Beta/3(qS) -> Body Frame F & M/3(qs)
  Alpha/Beta/4(Speed) -> Body Frame F & M/4(Airspeed), Airspeed/1
  "df, deg"/1 -> Body Frame F & M/9("df, deg")
  p,q,r/1 -> Body Frame F & M/10(p,q,r)
  Alpha/Beta/2("beta, deg") -> Body Frame F & M/2("Beta, deg")
  "dr, deg"/1 -> Body Frame F & M/8("dr, deg")
  daL,deg/1 -> Body Frame F & M/6("daL, deg")
  Alpha/Beta/1("alpha, deg") -> Body Frame F & M/1("Alpha, deg")
  "de, deg"/1 -> Body Frame F & M/5("de, deg")
  "Wind {E}"/1 -> Vair/2
  daR,deg/1 -> Body Frame F & M/7("daR, deg")

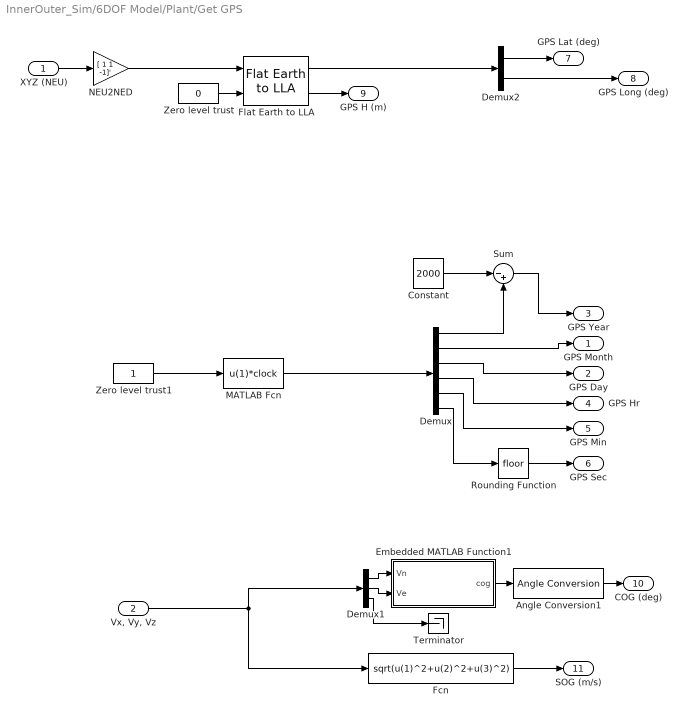
== system InnerOuter_Sim/6DOF Model/Plant/Get GPS ==
  XYZ (NEU) : Inport
  "Vx, Vy, Vz" : Inport  Port=2
  Angle Conversion1 : aerolibconvert2/Angle Conversion  SystemSampleTime=-1  IU=rad  OU=deg
  Constant : Constant  Value=2000
  Demux : Demux  Outputs=6
  Demux1 : Demux  Outputs=3
  Demux2 : Demux  Outputs=2
  Embedded MATLAB Function1 : Stateflow chart
  Fcn : Fcn  Expr=sqrt(u(1)^2+u(2)^2+u(3)^2)
  Flat Earth to LLA : aerolibtransform2/Flat Earth to LLA  SystemSampleTime=-1  units=Metric (MKS)  ptype=Earth (WGS84)  F=1/298.257223563  R=6378137  LL0=[37.0004768371582, -122.061897277832]  psi=0
  MATLAB Fcn : MATLABFcn  MATLABFcn=u(1)*clock  OutputSignalType=real  SampleTime=SampleT
  NEU2NED : Gain  Gain=[ 1 1 -1]'  SaturateOnIntegerOverflow=on
  Rounding Function : Rounding
  Sum : Sum  Inputs=|-+
  Terminator : Terminator
  Zero level trust : Constant  Value=0  SampleTime=SampleT
  Zero level trust1 : Constant  SampleTime=SampleT
  GPS Month : Outport
  GPS Day : Outport  Port=2
  GPS Year : Outport  Port=3
  GPS Hr : Outport  Port=4
  GPS Min : Outport  Port=5
  GPS Sec : Outport  Port=6
  GPS Lat (deg) : Outport  Port=7
  GPS Long (deg) : Outport  Port=8
  GPS H (m) : Outport  Port=9
  COG (deg) : Outport  Port=10
  SOG (m/s) : Outport  Port=11
  wires:
  NEU2NED/1 -> Flat Earth to LLA/1
  Zero level trust/1 -> Flat Earth to LLA/2
  XYZ (NEU)/1 -> NEU2NED/1
  Flat Earth to LLA/1 -> Demux2/1
  Flat Earth to LLA/2 -> GPS H (m)/1
  Zero level trust1/1 -> MATLAB Fcn/1
  MATLAB Fcn/1 -> Demux/1
  Demux/2 -> GPS Month/1
  Demux/3 -> GPS Day/1
  Demux/4 -> GPS Hr/1
  Demux/5 -> GPS Min/1
  Demux/6 -> Rounding Function/1
  Rounding Function/1 -> GPS Sec/1
  Demux2/1 -> GPS Lat (deg)/1
  Demux2/2 -> GPS Long (deg)/1
  Fcn/1 -> SOG (m/s)/1
  Demux1/1 -> Embedded MATLAB Function1/1(Vn)
  Demux1/2 -> Embedded MATLAB Function1/2(Ve)
  "Vx, Vy, Vz"/1 -> Demux1/1, Fcn/1
  Embedded MATLAB Function1/1(cog) -> Angle Conversion1/1
  Angle Conversion1/1 -> COG (deg)/1
  Demux/1 -> Sum/2
  Constant/1 -> Sum/1
  Sum/1 -> GPS Year/1
  Demux1/3 -> Terminator/1

== system InnerOuter_Sim/6DOF Model/Plant/ISA Atmosphere & Winds ==
  "X, Y, Z" : Inport
  Euler : Inport  Port=2
  Wind On : Inport  Port=3
  Airspeed : Inport  Port=4
  Add : Sum  Inputs=2  OutScaling=2^-10
  Constant : Constant  Value=[ 0 0 0]
  Dryden Wind Turbulence Model  (Discrete (+q -r)) : aerolibwind2/Dryden Wind Turbulence Model  (Continuous (+q -r))  SystemSampleTime=-1  units=Metric (MKS)  spec=MIL-F-8785C  model=Discrete Dryden (+q -r)  W20=windBase*0.3  Wdeg=windDirTurb  TurbProb=10^-2 - Light  L_high=533.4  Wingspan=span  ts=0.005  Seed=[23341 23342 23343 23344]  T_on=on
  Euler Angles to  Direction Cosine Matrix : aerolibtransform2/Euler Angles to  Direction Cosine Matrix  SystemSampleTime=-1
  Get Z : Selector  IndexOptions=Index vector (dialog)  Indices=[3]  OutputSizes=[(-2)]  InputPortWidth=3
  Horizontal Wind Model : aerolibwind2/Horizontal Wind Model  SystemSampleTime=-1  units=Metric (MKS)  Vw_source=Internal  Vwind=windBase  W_source=Internal  Wdeg=windDirHor
  ISA Atmosphere Model1 : aerolibatmos2/ISA Atmosphere Model  SystemSampleTime=-1  custom=off  g=9.80665  gamma=1.4  R=287.0531  L=0.0065  h_trop=11000  h_strat=20000  rho0=1.225  P0=101325  T0=288.15
  Reduce Z Wind : Gain  Gain=[1 1 0.1]
  Rotate to E Frame : Product  Multiplication=Matrix(*)
  Scope : Scope
      settings: YMin=-1  YMax=13  SaveName=windData  DataFormat=Array
  Switch : Switch  Criteria=u2 > Threshold  Threshold=0.3
  Terminator1 : Terminator
  Transpose : dspmtrx3/Transpose  SystemSampleTime=-1  Hermitian=off  overflowFlag=off
  Unit Delay : UnitDelay  SampleTime=-1
  Rho : Outport
  "Wind, {E}" : Outport  Port=2
  AirPressure (Pa) : Outport  Port=3
  OAT (K) : Outport  Port=4
  wires:
  "X, Y, Z"/1 -> Get Z/1
  Get Z/1 -> ISA Atmosphere Model1/1, Dryden Wind Turbulence Model  (Discrete (+q -r))/1
  ISA Atmosphere Model1/4 -> Rho/1
  ISA Atmosphere Model1/1 -> OAT (K)/1
  ISA Atmosphere Model1/2 -> Terminator1/1
  ISA Atmosphere Model1/3 -> AirPressure (Pa)/1
  Euler/1 -> Euler Angles to  Direction Cosine Matrix/1
  Euler Angles to  Direction Cosine Matrix/1 -> Dryden Wind Turbulence Model  (Discrete (+q -r))/3, Horizontal Wind Model/1, Transpose/1  "RECEF2B"
  Airspeed/1 -> Unit Delay/1
  Add/1 -> Switch/1
  Unit Delay/1 -> Dryden Wind Turbulence Model  (Discrete (+q -r))/2
  Horizontal Wind Model/1 -> Add/2
  Switch/1 -> Rotate to E Frame/2
  Wind On/1 -> Switch/2
  Constant/1 -> Switch/3
  Transpose/1 -> Rotate to E Frame/1
  Rotate to E Frame/1 -> "Wind, {E}"/1, Scope/1
  Dryden Wind Turbulence Model  (Discrete (+q -r))/1 -> Reduce Z Wind/1
  Reduce Z Wind/1 -> Add/1

== system InnerOuter_Sim/6DOF Model/Plant/Magnetometer ==
  Euler : Inport
  LTP2B : dspmtrx3/Transpose  SystemSampleTime=-1  Hermitian=off  overflowFlag=off
  Mag Field in nT source:  http://www.ngdc.noaa.gov/geomagmodels/struts/calcIGRFWMM : Constant  Value=magField
  Product : Product  Multiplication=Matrix(*)  RndMeth=Zero
  RB2LTP : Subsystem
  "Mag, nT" : Outport
  wires:
  RB2LTP/1(Rot) -> LTP2B/1
  LTP2B/1 -> Product/1
  Mag Field in nT source:  http://www.ngdc.noaa.gov/geomagmodels/struts/calcIGRFWMM/1 -> Product/2
  Euler/1 -> RB2LTP/1(Euler)
  Product/1 -> "Mag, nT"/1

== system InnerOuter_Sim/6DOF Model/Plant/[0, pi] Wrap Around ==
  Euler : Inport
  Compare To Zero : simulink/Logic and Bit Operations/Compare To Zero  SystemSampleTime=-1  relop=>=  LogicOutDataTypeMode=uint8  ZeroCross=off
  Logical Operator : Logic  Operator=NOT  AllPortsSameDT=off  OutDataTypeMode=Boolean
  Merge : Merge
  Mux2 : Mux  Inputs=2
  Negative Yaw : Subsystem
  Positive Yaw : Subsystem
  Selector1 : Selector  IndexOptions=Index vector (dialog)  Indices=[1 2]  OutputSizes=1  InputPortWidth=3
  Selector2 : Selector  IndexOptions=Index vector (dialog)  Indices=[3]  OutputSizes=1  InputPortWidth=3
  Euler-Wrapped : Outport
  wires:
  Euler/1 -> Selector2/1, Selector1/1
  Selector1/1 -> Mux2/1
  Mux2/1 -> Euler-Wrapped/1
  Selector2/1 -> Compare To Zero/1, Positive Yaw/1(yaw), Negative Yaw/1(yaw)
  Compare To Zero/1 -> Positive Yaw/Enable, Logical Operator/1
  Logical Operator/1 -> Negative Yaw/Enable
  Merge/1 -> Mux2/2
  Positive Yaw/1(yaw_wr) -> Merge/1
  Negative Yaw/1(yaw_wr) -> Merge/2

== system InnerOuter_Sim/6DOF Model/Split Ailerons And Introduce Failures/Aileron Flaping Failure ==
  Pulse Generator1 : DiscretePulseGenerator  PulseType=Time based  Amplitude=da_failamp  Period=da_failper  PulseWidth=50
  Vair2 : Sum  Inputs=+++  SaturateOnIntegerOverflow=on  InputSameDT=on
  da_failbias : Constant  Value=da_failbias
  da_failbias1 : Constant  Value=0
  "da, Fail, deg" : Outport
  wires:
  Pulse Generator1/1 -> Vair2/1
  da_failbias/1 -> Vair2/2
  da_failbias1/1 -> Vair2/3
  Vair2/1 -> "da, Fail, deg"/1

== system InnerOuter_Sim/6DOF Model/Split Ailerons And Introduce Failures/Rudder Failure ==
  Pulse Generator1 : DiscretePulseGenerator  PulseType=Time based  Amplitude=dr_failamp  Period=dr_failper  PulseWidth=50
  Vair2 : Sum  Inputs=+++  SaturateOnIntegerOverflow=on  InputSameDT=on
  da_failbias : Constant  Value=dr_failbias
  da_failbias1 : Constant  Value=0
  "da, Fail, deg" : Outport
  wires:
  Vair2/1 -> "da, Fail, deg"/1
  da_failbias1/1 -> Vair2/3
  da_failbias/1 -> Vair2/2
  Pulse Generator1/1 -> Vair2/1

== system InnerOuter_Sim/BaroTest/Initial Baro Bias/Low Pass8 ==
  In1 : Inport
  Discrete Zero-Pole : DiscreteZeroPole  Zeros=zerosd  Poles=polesd  Gain=gaind  SampleTime=SampleTime
  Out1 : Outport
  wires:
  In1/1 -> Discrete Zero-Pole/1
  Discrete Zero-Pole/1 -> Out1/1

== system InnerOuter_Sim/L1 Output Feedback Controller With  Projection Operator/Control  Law/Compute Coef ==
  a : Inport
  Enable : EnablePort
  -T : Gain  Gain=-apSampleTime  SampleTime=apSampleTime
  1-c : Sum  Inputs=-+  OutDataTypeMode=single  OutScaling=2^-10  SampleTime=apSampleTime
  Constant : Constant
  Subsystem11 : Subsystem  AncestorBlock=SLUGS_Library/Subsystem11
  b : Outport
  c : Outport  Port=2
  wires:
  a/1 -> -T/1
  1-c/1 -> b/1
  Constant/1 -> 1-c/2
  Subsystem11/1(exp(u)) -> c/1, 1-c/1  "c"
  -T/1 -> Subsystem11/1(u)

== system InnerOuter_Sim/L1 Output Feedback Controller With  Projection Operator/Control  Law/Detect Change ==
  Data : Inport
  Abs1 : Abs  SampleTime=apSampleTime
  Difference1 : simulink/Discrete/Difference  SystemSampleTime=-1  ICPrevInput=0.0  OutDataType=sfix(16)  OutScaling=2^-10  DoSatur=off
  Saturation1 : Saturate  UpperLimit=1  LowerLimit=0  SampleTime=apSampleTime
  change? : Outport
  wires:
  Saturation1/1 -> change?/1
  Data/1 -> Difference1/1
  Abs1/1 -> Saturation1/1
  Difference1/1 -> Abs1/1

== system InnerOuter_Sim/L1 Output Feedback Controller With  Projection Operator/Projection Operator/Enabled Subsystem ==
  In1 : Inport
  Enable : EnablePort
  Out1 : Outport
  wires:
  In1/1 -> Out1/1

== system InnerOuter_Sim/L1 Output Feedback Controller With  Projection Operator/Projection Operator/Enabled Subsystem1 ==
  y : Inport
  f_the : Inport  Port=2
  grad : Inport  Port=3
  Enable : EnablePort
  Constant : Constant  OutDataTypeMode=single
  Divide1 : Product  OutDataTypeMode=single  OutScaling=2^-10
  Divide2 : Product  OutDataTypeMode=single  OutScaling=2^-10
  Sign : Signum
  Subtract : Sum  Inputs=+-  OutDataTypeMode=single  OutScaling=2^-10
  Out1 : Outport
  wires:
  Divide2/1 -> Out1/1
  y/1 -> Divide2/1
  Subtract/1 -> Divide2/2
  f_the/1 -> Divide1/1
  Constant/1 -> Subtract/1
  Sign/1 -> Divide1/2
  grad/1 -> Sign/1
  Divide1/1 -> Subtract/2

== system InnerOuter_Sim/L1 Output Feedback Controller With  Projection Operator/Projection Operator/Enabled Subsystem2 ==
  y : Inport
  f_the : Inport  Port=2
  grad : Inport  Port=3
  Enable : EnablePort
  Constant : Constant  OutDataTypeMode=single
  Divide1 : Product  OutDataTypeMode=single  OutScaling=2^-10
  Divide2 : Product  OutDataTypeMode=single  OutScaling=2^-10
  Sign : Signum
  Subtract : Sum  Inputs=+-  OutDataTypeMode=single  OutScaling=2^-10
  Out1 : Outport
  wires:
  Divide1/1 -> Subtract/2
  grad/1 -> Sign/1
  Sign/1 -> Divide1/2
  Constant/1 -> Subtract/1
  f_the/1 -> Divide1/1
  Subtract/1 -> Divide2/2
  y/1 -> Divide2/1
  Divide2/1 -> Out1/1

== system InnerOuter_Sim/L1 Output Feedback Controller With  Projection Operator/Projection Operator/F(theta) ==
  Theta Max : Inport
  Eps 0 : Inport  Port=2
  Theta : Inport  Port=3
  Constant : Constant  Value=2  OutDataTypeMode=single
  Divide : Product  OutDataTypeMode=single  OutScaling=2^-10
  Divide1 : Product  OutDataTypeMode=single  OutScaling=2^-10
  Divide2 : Product  OutDataTypeMode=single  OutScaling=2^-10
  Divide3 : Product  Inputs=*/  OutDataTypeMode=single  OutScaling=2^-10
  Divide4 : Product  Inputs=/**  OutDataTypeMode=single  OutScaling=2^-10
  Subtract : Sum  Inputs=+-  OutDataTypeMode=single  OutScaling=2^-10
  "Theta " : InportShadow  Port=3  LatchByCopyingInsideSignal=off
  f_theta : Outport
  dif_f_theta : Outport  Port=2
  wires:
  Divide4/1 -> dif_f_theta/1
  "Theta "/1 -> Divide4/2
  Constant/1 -> Divide4/3
  Divide3/1 -> f_theta/1
  Divide2/1 -> Divide4/1, Divide3/2
  Subtract/1 -> Divide3/1
  Eps 0/1 -> Divide2/2
  Divide1/1 -> Divide2/1, Subtract/2
  Divide/1 -> Subtract/1
  Theta Max/1 -> Divide1/1, Divide1/2
  Theta/1 -> Divide/2, Divide/1
